simulink model "TrackerSimulation"  (R2021a)
settings: Solver=FixedStepAuto  StartTime=0.0  StopTime=inf  RelTol=1e-3  EnableMultiTasking=on
settings Model: SimulationMode=accelerator  SILPILModeSetting=veronly  EnablePacing=on  ExtModeTrigDuration=2  Creator=cstap  LastModifiedBy=Goblin
settings SolverCC: AlgebraicLoopSolver=TrustRegion  AutoInsertRateTranBlk=on
settings OptimizationCC: EnhancedBackFolding=on  PassReuseOutputArgsAs=Individual arguments  ZeroExternalMemoryAtStartup=off  ZeroInternalMemoryAtStartup=off  MaxStackSize=64  OptimizeBlockOrder=speed  DifferentSizesBufferReuse=on  OptimizationCustomize=off  EfficientTunableParamExpr=on
settings DebuggingCC: ParameterTunabilityLossMsg=error  SFMachineParentedDataDiag=warning
settings HardwareCC: ProdBitPerInt=16  ProdBitPerPointer=16  ProdBitPerSizeT=16  ProdBitPerPtrDiffT=16  ProdLargestAtomicFloat=None  ProdWordSize=8  ProdHWDeviceType=Atmel->AVR  UseEmbeddedCoderFeatures=off
settings SFSimCC: MATLABDynamicMemAlloc=off
settings RTWCC: SystemTargetFile=ert.tlc  HardwareBoard=Arduino Uno  TemplateMakefile=ert_default_tmf  Toolchain=Arduino AVR  BuildConfiguration=Faster Runs
settings CodeAppCC: ForceParamTrailComments=on  IgnoreCustomStorageClasses=off  OperatorAnnotations=on  SimulinkDataObjDesc=on  SFDataObjDesc=on  InsertBlockDesc=on
settings ERTTargetCC: SupportContinuousTime=on  SupportNonInlinedSFcns=on  SupportVariableSizeSignals=on  ExtModeStaticAllocSize=250

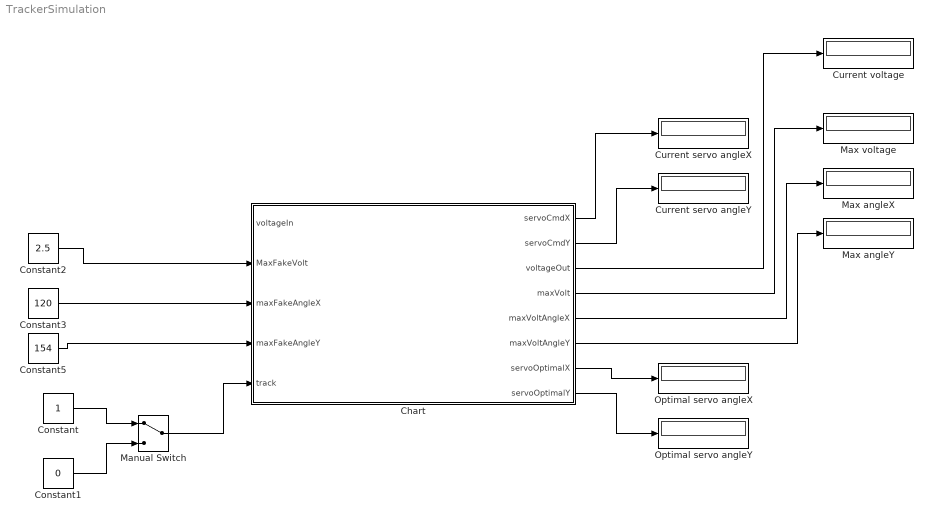
== system TrackerSimulation ==
  Chart : Stateflow chart  TreatAsAtomicUnit=on
      settings: PortSchema="{\"entries\":[{\"content\":{\"sides\":[{\"content\":{\"connectorIds\":[\"In2\",\"In3\",\"In5\",\"In4\",\"In1\"]},\"type\":\"ConnectorPlacement.EquallySpacedRectSide\",\"uuid\":\"8b860831-5c3c-424c-9ef6-047f14fc176a\"},{\"content\":{\"connectorIds\":[\"Out3\",\"Out2\",\"Out4\",\"Out5\",\"Out1\",\"Out6\",\"Out7\",\"Out8\"],\"side\":\"RIGHT\"},\"type\":\"ConnectorPlacement.EquallySpacedRectSide\",\"uuid\":\"17905b88-ecc9-49a7-8549-0f05587c3ec9\"},{\"content\":{\"connectorIds\":[],\"side\":\"TOP\"},\"type\":\"ConnectorPlacement.EquallySpacedRectSide\",\"uuid\":\"4ee64023-cfd9-4168-9375-d64fa3cfec3e\"}]},\"type\":\"ConnectorPlacement.EquallySpacedConnector\",\"uuid\":\"090b8424-d4f1-4d97-9e98-1b13f24abbbb\"}],\"packageUris\":[\"http://schema.mathworks.com/mf0/Connector/R2020b\"],\"version\":\"1.0\"}"
  Constant : Constant
  Constant1 : Constant  Value=0
  Constant2 : Constant  Value=2.5
  Constant3 : Constant  Value=120
  Constant5 : Constant  Value=154
  Current servo angleX : Display
  Current servo angleY : Display
  Current voltage : Display
  Manual Switch : ManualSwitch
  Max angleX : Display
  Max angleY : Display
  Max voltage : Display
  Optimal servo angleX : Display
  Optimal servo angleY : Display
  wires:
  Chart/5(maxVolt) -> Max voltage/1
  Constant/1 -> Manual Switch/1
  Constant1/1 -> Manual Switch/2
  Manual Switch/1 -> Chart/1(track)
  Chart/4(voltageOut) -> Current voltage/1
  Chart/3(servoCmdX) -> Current servo angleX/1
  Chart/1(maxVoltAngleX) -> Max angleX/1
  Constant2/1 -> Chart/3(MaxFakeVolt)
  Constant3/1 -> Chart/5(maxFakeAngleX)
  Constant5/1 -> Chart/4(maxFakeAngleY)
  Chart/6(maxVoltAngleY) -> Max angleY/1
  Chart/2(servoCmdY) -> Current servo angleY/1
  Chart/7(servoOptimalX) -> Optimal servo angleX/1
  Chart/8(servoOptimalY) -> Optimal servo angleY/1

== stateflow chart TrackerSimulation/Chart ==
  settings: updateMethod=DISCRETE  sampleTime=0.1
  state Wait
  state ScanAndGoToMaxVoltage
    state ResetPosition
      maxVolt = 0;
      maxVoltAngleX = 0;
      maxVoltAngleY = 0;
      servoCmdX =  0;
      servoCmdY = 0;
      voltage = 0;
    state Increment1
      entry: i = i + 1;
    state Increment
      entry: i = i + 1;
    state ScanVoltagesX
      servoCmdX = angleRange(i);
      %voltage = voltageIn;
      voltage = MaxFakeVolt/3*(3-abs(servoCmdX-maxFakeAngleX)/180-abs(servoCmdY-maxFakeAngleY)/180);%fake input
      if voltage > maxVolt
      maxVolt=voltage;
      maxVoltAngleX = angleRange(i)
      end
      voltageOut = voltage;
    state ScanVoltagesY
      servoCmdY = angleRange(i);
      %voltage = voltageIn;
      voltage = MaxFakeVolt/3*(3-abs(servoCmdX-maxFakeAngleX)/180-abs(servoCmdY -maxFakeAngleY)/180);%fake input
      if voltage > maxVolt
      maxVolt=voltage;
      maxVoltAngleY = angleRange(i);
      end
      voltageOut = voltage;
    state GoToMaxVoltageX
      servoCmdX = maxVoltAngleX;
      maxVolt = 0;
    state CheckNearAnglesX
      checkAgain=false;
      testServoCmdX=servoCmdX + 1;
      if testServoCmdX < 181
      servoCmdX = testServoCmdX;
      pause(0.5);
      end
      %voltage = voltageIn
      voltage = MaxFakeVolt/3*(3-abs(servoCmdX-maxFakeAngleX)/180-abs(servoCmdY -maxFakeAngleY)/180);%fake input
      if voltage > maxVolt
      checkAgain=true;
      maxVoltAngleX=servoCmdX;
      maxVolt = voltage;
      else
      testServoCmdX=testServoCmdX-2;
      if testServoCmdX > 0
      servoCmdX=testServoCmdX;
      pause(0.5);
      end
      %voltage = voltageIn
      voltage = MaxFakeVolt/3*(3-abs(servoCmdX-maxFakeAngleX)/180-abs(servoCmdY -maxFakeAngleY)/180);%fake input
      if voltage > maxVolt
      checkAgain=true;
      maxVoltAngleX=servoCmdX;
      maxVolt = voltage;
      else
      servoCmdX = testServoCmdX +1;
      pause(0.5);
      end
      end
    state GoToMaxVoltageY
      servoCmdY  = maxVoltAngleY;
    state NewMaxVoltage
      maxVolt=voltage;
    state IsVoltageChanged
      servoOptimalX=servoCmdX;
      servoOptimalY=servoCmdY;
      %voltage = voltageIn;
      voltage = MaxFakeVolt/3*(3-abs(servoCmdX-maxFakeAngleX)/180-abs(servoCmdY -maxFakeAngleY)/180);%fake input
      voltageOut = voltage;
      if voltage > maxVolt
      maxVolt = voltage;
      end
      dif=voltage-maxVolt;
    state CheckNearAnglesY
      checkAgain=false;
      testServoCmdY=servoCmdY + 1;
      if testServoCmdY < 181
      servoCmdY = testServoCmdY;
      pause(0.5);
      end
      %voltage = voltageIn
      voltage = MaxFakeVolt/3*(3-abs(servoCmdX-maxFakeAngleX)/180-abs(servoCmdY -maxFakeAngleY)/180);%fake input
      if voltage > maxVolt
      checkAgain=true;
      maxVoltAngleY=servoCmdY;
      maxVolt = voltage;
      else
      testServoCmdY=testServoCmdY-2;
      if testServoCmdY > 0
      servoCmdY=testServoCmdY;
      pause(0.5);
      end
      %voltage = voltageIn
      voltage = MaxFakeVolt/3*(3-abs(servoCmdX-maxFakeAngleX)/180-abs(servoCmdY -maxFakeAngleY)/180);%fake input
      if voltage > maxVolt
      checkAgain=true;
      maxVoltAngleY=servoCmdY;
      maxVolt = voltage;
      else
      servoCmdY = testServoCmdY +1;
      pause(0.5);
      end
      end
    (default) -> ResetPosition : {angleRange = 0  :180;}
    Increment1 -> ScanVoltagesY : after(0.01,sec)
    ScanVoltagesY -> Increment1 [order 1] : [i < 181]
    Increment -> ScanVoltagesX : after(0.01,sec)
    ScanVoltagesX -> Increment [order 1] : [i < 181]
    ResetPosition -> ScanVoltagesX : {i = 1;}
    ScanVoltagesX -> GoToMaxVoltageX [order 2] : after(2,sec)[i==181]{i = 1;}
    GoToMaxVoltageX -> ScanVoltagesY : after(2,sec)
    ScanVoltagesY -> GoToMaxVoltageY [order 2] : after(2,sec)[i==181]
    CheckNearAnglesX -> CheckNearAnglesX [order 1] : [checkAgain == true]
    NewMaxVoltage -> CheckNearAnglesX
    IsVoltageChanged -> NewMaxVoltage [order 2] : [dif<0]
    GoToMaxVoltageY -> IsVoltageChanged : after(2,sec)
    IsVoltageChanged -> IsVoltageChanged [order 1] : after(2,sec)[dif >=0]
    CheckNearAnglesX -> CheckNearAnglesY [order 2] : [checkAgain==false]
    CheckNearAnglesY -> IsVoltageChanged [order 2] : [checkAgain==false]
    CheckNearAnglesY -> CheckNearAnglesY [order 1] : [checkAgain==true]
  (default) -> Wait
  Wait -> ScanAndGoToMaxVoltage : [track==1]
  ScanAndGoToMaxVoltage -> Wait : [track==0]
  data: i local; angleRange local; track input; maxVoltAngleX output; servoCmdY output; dif local; voltageIn input; servoCmdX output; voltageOut output; voltage local; maxVolt output; MaxFakeVolt input; maxFakeAngleY input; maxFakeAngleX input; maxVoltAngleY output; checkAgain local; testServoCmdY local; testServoCmdX local; servoOptimalX output; servoOptimalY output
